simulink model "soce"  (R2024a)
settings: Solver=VariableStepAuto  StartTime=0.0  StopTime=10  FixedStep=500e-6  RelTol=1e-3
values from neighbouring files (symbols this model uses):
  C1_pack = C1 * parallel_cells / series_cells    (= 0.0780484375)    [soc.m]
  C2_pack = C2 * parallel_cells / series_cells    (= 0.0972984375)    [soc.m]
  internal_resistance_pack = int_cell_resistance * series_cells / parallel_cells + electronic_resistance    (= 0.104737272727)    [soc.m]
  Q_2RC = 1    [soc.m]
  R = [sigma_V^2, 0 ... (first row only)    [soc.m]
  R1_pack = R1 * series_cells / parallel_cells    (= 0.0116363636364)    [soc.m]
  R2_pack = R2 * series_cells / parallel_cells    (= 0.0116363636364)    [soc.m]
undefined symbols (not defined in the file or in its folder): rated_cell_capacity, T_vec
libraries: simulink x10, spsVariableCapacitorLib x3, spsVariableResistorLib x3, spsCurrentMeasurementLib x2, spsVoltageMeasurementLib x2, spsControlledVoltageSourceLib x1, spsControlledCurrentSourceLib x1, sps_lib x1
settings Model: Creator=DELL  LastModifiedBy=DELL

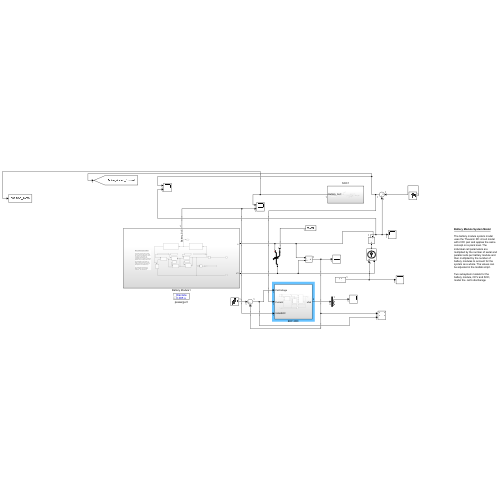
[thumbnail: Simulink's stored preview of the top-level diagram]
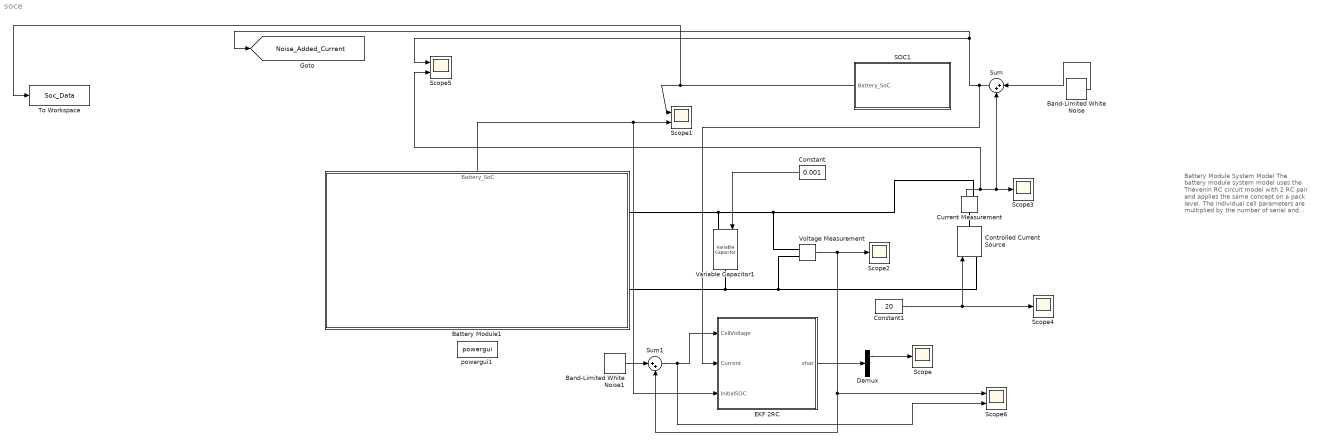
== system soce ==
  note: Battery Module System Model
      |
      | The battery module system model uses the Thevenin RC circuit model with 2 RC pair and applies the same concept on a pack level. The individual cell parameters are multiplied by the number of serial and parallel cells per battery module and then multiplied by the number of battery module s to account for the system as a whole. The values can be adjusted in the matlab script.
      |
      | Two subsystem models for the battery module , OCV and SOC, model the cell's discharage characteristic and state of charge for the ESUs.
  Band-Limited White Noise : simulink/Sources/Band-Limited White Noise  Cov=0  Ts=1  seed=12345
  Band-Limited White Noise1 : simulink/Sources/Band-Limited White Noise  Cov=0  Ts=0.01  seed=12345
  Battery Module1 : Subsystem
      settings: PortSchema="{\"entries\":[{\"content\":{\"sides\":[{\"content\":{},\"type\":\"ConnectorPlacement.EquallySpacedRectSide\",\"uuid\":\"1cf2e637-c056-448b-9d8f-ed664b461c4e\"},{\"content\":{\"connectorIds\":[\"RConn1\",\"RConn2\"],\"side\":\"RIGHT\"},\"type\":\"ConnectorPlacement.EquallySpacedRectSide\",\"uuid\":\"9015fd1e-0347-435a-aa67-edb519119c95\"},{\"content\":{\"connectorIds\":[\"Out1\"],\"side\":\"TOP\"},\"type\":\"ConnectorPlacement.EquallySpacedRectSide\",\"uuid\":\"8eddc867-8dee-40eb-ad4a-8474d27a660f\"}]},\"type\":\"ConnectorPlacement.EquallySpacedConnector\",\"uuid\":\"c8be1dcd-ca4d-45ed-81e7-8f26517ac315\"}],\"packageUris\":[\"http://schema.mathworks.com/mf0/Connector/R2020b\"],\"version\":\"1.0\"}"
  Constant : Constant  Value=0.001
  Constant1 : Constant  Value=20
  Controlled Current Source : spsControlledCurrentSourceLib/Controlled Current Source  Initialize=on  Source_Type=AC  Amplitude=0  Phase=0  Frequency=0  Measurements=None
  Current Measurement : spsCurrentMeasurementLib/Current Measurement  PhasorSimulation=off  OutputType=Complex  PSBequivalent=0
  Demux : Demux  Outputs=3
  EKF 2RC : Subsystem  VariantControl=EKF 2RC
      settings: LibrarySourceBlock=|
      | BatteryEstimators/SOC Estimator
      | (Kalman Filter)/Kalman Filter/EKF 2RC
  SOC1 : Subsystem
  Scope{,2..4} (4 alike) : Scope
  Scope1 : Scope  NumInputPorts=2
  Scope5 : Scope  NumInputPorts=2
  Scope6 : Scope  NumInputPorts=2
  Sum : Sum  Inputs=|++
  Sum1 : Sum  Inputs=|++
  To Workspace : ToWorkspace  VariableName=Soc_Data  SaveFormat=Timeseries  SampleTime=-1
  Variable Capacitor1 : spsVariableCapacitorLib/Variable Capacitor  methode=Backward Euler  Cabsmin=1e-9  Initialize=on  vC0=0.001  C0=1e-6  iC0=0
      settings: LibrarySourceBlock=sps_lib/Passives/Variable Capacitor
  Voltage Measurement : spsVoltageMeasurementLib/Voltage Measurement  PhasorSimulation=off  OutputType=Complex  PSBequivalent=0
  powergui1 : sps_lib/powergui  SimulationMode=Discrete  SampleTime=0.005  frequency=60  Iterations=50  frequencyindice=0  Pbase=100e6  ErrMax=1e-4  UnitsV=kV  UnitsW=MW  buscounter=0  FunctionMessages=off  echomessages=off  EnableUseOfTLC=off  CurrentSourceSwitches=off  DisableSnubberDevices=off  DisableRonSwitches=off  DisableVfSwitches=off  DisplayEquations=off  AutomaticDiscreteSolvers=off  SolverType=Tustin  Interpol=off  ExternalGateDelay=off  methode=off  Ts=0  x0status=blocks  SPID=off  SwTol=0  HookPort=off  NonlinearTolerance=1e-4  nMaxIteration=100  ContinueOnMaxIteration=off  RestoreLinks=warning  ResistiveCurrentMeasurement=off  Frange=[0:2:500]  Ylog=off  Xlog=on  ShowGrid=off  save=off  variable=ZData  structure=0  ZoomFFT=on  StartTime=0.0  cycles=1  DisplayStyle=1  fundamental=60  FreqAxis=off  MaxFrequency=1000  frequencyindicesteady=1  RmsSteady=1  display=off
  tag scope: Noise_Added_Current=global
  wires:
  Band-Limited White Noise/1 -> Sum/1
  SOC1/1(Battery_SoC) -> To Workspace/1, Scope1/1
  Constant/1 -> Variable Capacitor1/1
  Current Measurement/1 -> Scope3/1, Sum/2, Scope5/2
  Constant1/1 -> Scope4/1, Controlled Current Source/1
  Band-Limited White Noise1/1 -> Sum1/1
  Sum/1 -> EKF 2RC/2(Current), Scope5/1, [Noise_Added_Current]
  Voltage Measurement/1 -> Scope2/1, Sum1/2, Scope6/1
  Battery Module1/1(Battery_SoC) -> EKF 2RC/3(InitialSOC), Scope1/2
  Sum1/1 -> Scope6/2, EKF 2RC/1(CellVoltage)
  EKF 2RC/1(xhat) -> Demux/1
  Demux/1 -> Scope/1
  connections:
  Variable Capacitor1/LConn1 -- Battery Module1/RConn1 -- Voltage Measurement/LConn2 -- Current Measurement/RConn1
  Controlled Current Source/LConn1 -- Voltage Measurement/LConn1 -- Battery Module1/RConn2 -- Variable Capacitor1/RConn1
  Current Measurement/LConn1 -- Controlled Current Source/RConn1

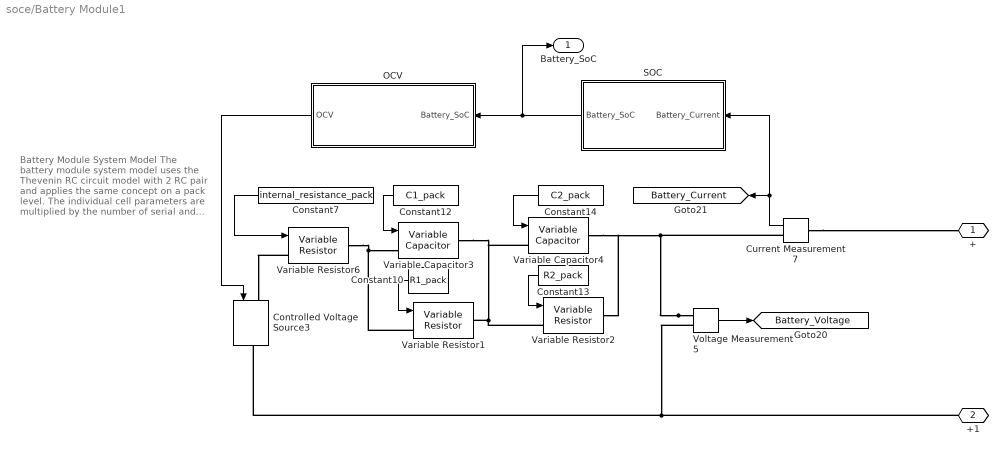
== system soce/Battery Module1 ==
  note: Battery Module System Model
      |
      | The battery module system model uses the Thevenin RC circuit model with 2 RC pair and applies the same concept on a pack level. The individual cell parameters are multiplied by the number of serial and parallel cells per battery module and then multiplied by the number of battery modules to account for the system as a whole. The values can be adjusted in the matlab script.
      |
      | Two subsystem models for the battery module, OCV and SOC, model the cell's discharage characteristic and state of charge for the ESUs.
  Constant10 : Constant  Value=R1_pack
  Constant12 : Constant  Value=C1_pack
  Constant13 : Constant  Value=R2_pack
  Constant14 : Constant  Value=C2_pack
  Constant7 : Constant  Value=internal_resistance_pack
  Controlled Voltage Source3 : spsControlledVoltageSourceLib/Controlled Voltage Source  Initialize=on  Source_Type=DC  Amplitude=537.6  Phase=0  Frequency=1  Measurements=None
  Current Measurement7 : spsCurrentMeasurementLib/Current Measurement  PhasorSimulation=off  OutputType=Complex  PSBequivalent=0
  OCV : Subsystem
  SOC : Subsystem
  Variable Capacitor3 : spsVariableCapacitorLib/Variable Capacitor  methode=Backward Euler  Cabsmin=1e-9  Initialize=off  vC0=4  C0=6  iC0=0
  Variable Capacitor4 : spsVariableCapacitorLib/Variable Capacitor  methode=Backward Euler  Cabsmin=1e-9  Initialize=off  vC0=0  C0=1100e-3  iC0=0
  Variable Resistor1 : spsVariableResistorLib/Variable Resistor  Rabsmin=1e-3
  Variable Resistor2 : spsVariableResistorLib/Variable Resistor  Rabsmin=1e-3
  Variable Resistor6 : spsVariableResistorLib/Variable Resistor  Rabsmin=1e-3
      settings: LibrarySourceBlock=sps_lib/Passives/Variable Resistor
  Voltage Measurement5 : spsVoltageMeasurementLib/Voltage Measurement  PhasorSimulation=off  OutputType=Complex  PSBequivalent=0
  + : PMIOPort  Side=Right
  +1 : PMIOPort  Port=2  Side=Right
  Battery_SoC : Outport
  tag scope: Battery_Current=global, Battery_Voltage=global
  wires:
  OCV/1(OCV) -> Controlled Voltage Source3/1
  Voltage Measurement5/1 -> [Battery_Voltage]
  Current Measurement7/1 -> SOC/1(Battery_Current), [Battery_Current]
  SOC/1(Battery_SoC) -> Battery_SoC/1, OCV/1(Battery_SoC)
  Constant14/1 -> Variable Capacitor4/1
  Constant7/1 -> Variable Resistor6/1
  Constant12/1 -> Variable Capacitor3/1
  Constant10/1 -> Variable Resistor1/1
  Constant13/1 -> Variable Resistor2/1
  connections:
  Variable Resistor2/LConn1 -- Variable Capacitor4/LConn1 -- Variable Capacitor3/RConn1 -- Variable Resistor1/RConn1
  Variable Resistor1/LConn1 -- Variable Resistor6/RConn1 -- Variable Capacitor3/LConn1
  Voltage Measurement5/LConn1 -- +1/RConn1 -- Controlled Voltage Source3/RConn1
  Variable Resistor6/LConn1 -- Controlled Voltage Source3/LConn1
  Voltage Measurement5/LConn2 -- Variable Resistor2/RConn1 -- Variable Capacitor4/RConn1 -- Current Measurement7/RConn1
  Current Measurement7/LConn1 -- +/RConn1

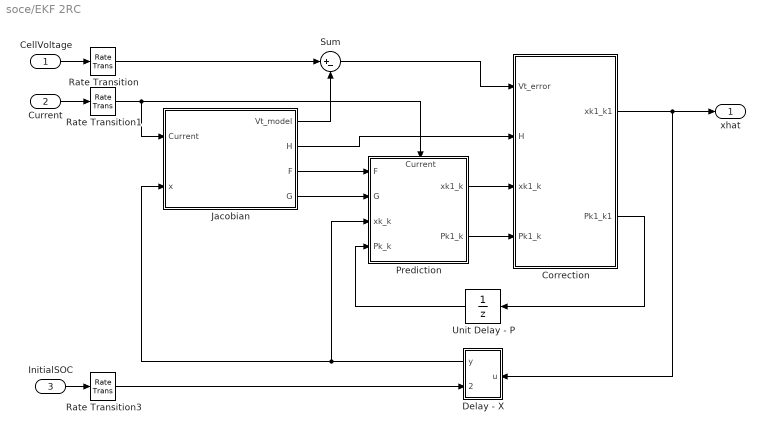
== system soce/EKF 2RC ==
  CellVoltage : Inport
  Current : Inport  Port=2
  InitialSOC : Inport  Port=3
  Correction : Subsystem
  Delay - X : Subsystem
      settings: PortSchema="{\"entries\":[{\"content\":{\"sides\":[{\"content\":{\"connectorIds\":[\"In1\"]},\"type\":\"ConnectorPlacement.EquallySpacedRectSide\",\"uuid\":\"3362b6e3-9ef0-414f-8c36-2f543f704d9c\"},{\"content\":{\"connectorIds\":[\"Out1\",\"In2\"],\"side\":\"RIGHT\"},\"type\":\"ConnectorPlacement.EquallySpacedRectSide\",\"uuid\":\"11e7d0c5-4a27-4b8c-b505-ab30596c2b25\"},{\"content\":{\"connectorIds\":[],\"side\":\"TOP\"},\"type\":\"ConnectorPlacement.EquallySpacedRectSide\",\"uuid\":\"2d2b4d79-d4b9-4064-9377-c3a75a280e90\"}]},\"type\":\"ConnectorPlacement.EquallySpacedConnector\",\"uuid\":\"61e54eb8-002c-4ced-aad8-a34ad65d09af\"}],\"packageUris\":[\"http://schema.mathworks.com/mf0/Connector/R2020b\"],\"version\":\"1.0\"}"
  Jacobian : Subsystem
  Prediction : Subsystem
      settings: PortSchema="{\"entries\":[{\"content\":{\"sides\":[{\"content\":{\"connectorIds\":[\"In1\",\"In2\",\"In3\",\"In4\"]},\"type\":\"ConnectorPlacement.EquallySpacedRectSide\",\"uuid\":\"769ad24d-2d7f-40f9-a049-32dd41bae35d\"},{\"content\":{\"connectorIds\":[\"Out1\",\"Out2\"],\"side\":\"RIGHT\"},\"type\":\"ConnectorPlacement.EquallySpacedRectSide\",\"uuid\":\"b91eca28-d625-4904-9292-6163fd48fb7b\"},{\"content\":{\"connectorIds\":[\"In5\"],\"side\":\"TOP\"},\"type\":\"ConnectorPlacement.EquallySpacedRectSide\",\"uuid\":\"03f245fa-72f0-4cdc-a162-c307173ac60c\"}]},\"type\":\"ConnectorPlacement.EquallySpacedConnector\",\"uuid\":\"70aef080-af31-4b50-8c38-7ffc1907abe4\"}],\"packageUris\":[\"http://schema.mathworks.com/mf0/Connector/R2020b\"],\"version\":\"1.0\"}"
  Rate Transition : RateTransition
  Rate Transition1 : RateTransition
  Rate Transition3 : RateTransition
  Sum : Sum  Inputs=|+-
  Unit Delay - P : UnitDelay  SampleTime=-1  HasFrameUpgradeWarning=on
  xhat : Outport
  wires:
  Current/1 -> Rate Transition1/1
  Prediction/1(xk1_k) -> Correction/3(xk1_k)
  Jacobian/1(Vt_model) -> Sum/2
  Rate Transition3/1 -> Delay - X/2(SOC0)
  CellVoltage/1 -> Rate Transition/1
  Rate Transition1/1 -> Prediction/5(Current), Jacobian/1(Current)
  Sum/1 -> Correction/1(Vt_error)
  Jacobian/4(G) -> Prediction/2(G)
  Correction/2(Pk1_k1) -> Unit Delay - P/1
  Delay - X/1(y) -> Prediction/3(xk_k), Jacobian/2(x)
  Prediction/2(Pk1_k) -> Correction/4(Pk1_k)
  Jacobian/2(H) -> Correction/2(H)
  Rate Transition/1 -> Sum/1
  Correction/1(xk1_k1) -> xhat/1, Delay - X/1(u)
  Unit Delay - P/1 -> Prediction/4(Pk_k)
  Jacobian/3(F) -> Prediction/1(F)
  InitialSOC/1 -> Rate Transition3/1

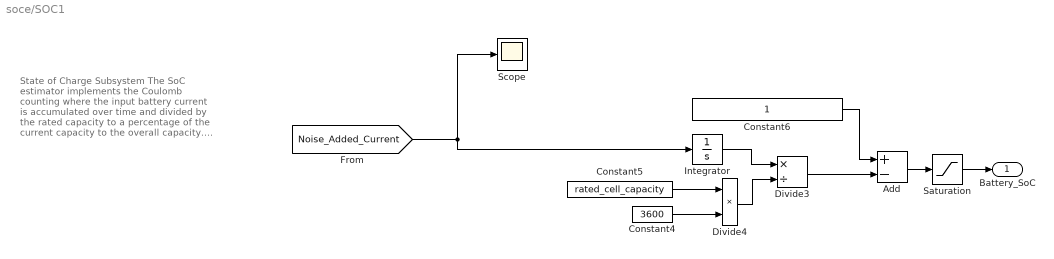
== system soce/SOC1 ==
  note: State of Charge Subsystem
      |
      | The SoC estimator implements the Coulomb counting where the input battery current is accumulated over time and divided by the rated capacity to a percentage of the current capacity to the overall capacity. The output of this subsystem outputs the state of charge as a percentage.
  Add : Sum  Inputs=+-
  Constant4 : Constant  Value=3600
  Constant5 : Constant  Value=rated_cell_capacity
  Constant6 : Constant
  Divide3 : Product  Inputs=*/
  Divide4 : Product  Inputs=**
  Integrator : Integrator
  Saturation : Saturate  UpperLimit=1  LowerLimit=0
  Scope : Scope
  Battery_SoC : Outport
  wires:
  Constant6/1 -> Add/1
  Divide3/1 -> Add/2
  Divide4/1 -> Divide3/2
  Constant5/1 -> Divide4/1
  Integrator/1 -> Divide3/1
  Constant4/1 -> Divide4/2
  [Noise_Added_Current] -> Integrator/1, Scope/1
  Saturation/1 -> Battery_SoC/1
  Add/1 -> Saturation/1

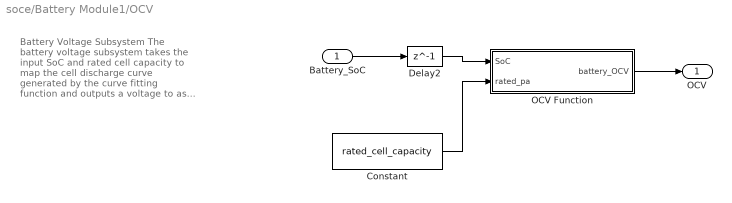
== system soce/Battery Module1/OCV ==
  note: Battery Voltage Subsystem
      |
      | The battery voltage subsystem takes the input SoC and rated cell capacity to map the cell discharge curve generated by the curve fitting function and outputs a voltage to as an input to the voltage source.
  Battery_SoC : Inport
  Constant : Constant  Value=rated_cell_capacity
  Delay2 : Delay  DelayLength=1  InitialCondition=1
  OCV Function : MATLAB Function  TreatAsAtomicUnit=on
  OCV : Outport
  wires:
  Delay2/1 -> OCV Function/1(SoC)
  OCV Function/1(battery_OCV) -> OCV/1
  Battery_SoC/1 -> Delay2/1
  Constant/1 -> OCV Function/2(rated_pa)

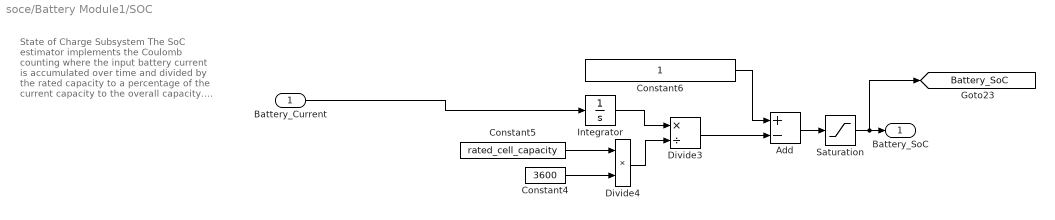
== system soce/Battery Module1/SOC ==
  note: State of Charge Subsystem
      |
      | The SoC estimator implements the Coulomb counting where the input battery current is accumulated over time and divided by the rated capacity to a percentage of the current capacity to the overall capacity. The output of this subsystem outputs the state of charge as a percentage.
  Battery_Current : Inport
  Add : Sum  Inputs=+-
  Constant4 : Constant  Value=3600
  Constant5 : Constant  Value=rated_cell_capacity
  Constant6 : Constant
  Divide3 : Product  Inputs=*/
  Divide4 : Product  Inputs=**
  Integrator : Integrator
  Saturation : Saturate  UpperLimit=1  LowerLimit=0
  Battery_SoC : Outport
  tag scope: Battery_SoC=global
  wires:
  Constant6/1 -> Add/1
  Divide3/1 -> Add/2
  Divide4/1 -> Divide3/2
  Constant5/1 -> Divide4/1
  Integrator/1 -> Divide3/1
  Constant4/1 -> Divide4/2
  Battery_Current/1 -> Integrator/1
  Saturation/1 -> [Battery_SoC], Battery_SoC/1
  Add/1 -> Saturation/1

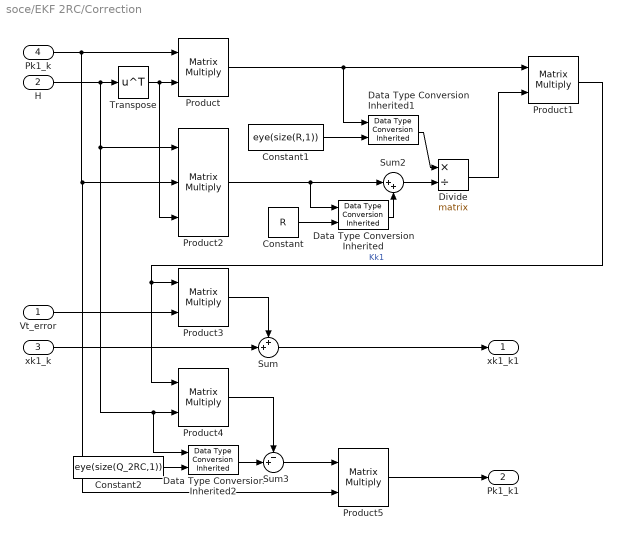
== system soce/EKF 2RC/Correction ==
  Vt_error : Inport
  H : Inport  Port=2
  xk1_k : Inport  Port=3
  Pk1_k : Inport  Port=4
  Constant : Constant  Value=R
  Constant1 : Constant  Value=eye(size(R,1))
  Constant2 : Constant  Value=eye(size(Q_2RC,1))
  Data Type Conversion Inherited : simulink/Signal Attributes/Data Type Conversion Inherited  ConvertRealWorld=Real World Value  DoSatur=off
  Data Type Conversion Inherited1 : simulink/Signal Attributes/Data Type Conversion Inherited  ConvertRealWorld=Real World Value  DoSatur=off
  Data Type Conversion Inherited2 : simulink/Signal Attributes/Data Type Conversion Inherited  ConvertRealWorld=Real World Value  DoSatur=off
  Divide : Product  Inputs=*/  Multiplication=Matrix(*)
  Product{,1,3..5} (5 alike) : Product  Multiplication=Matrix(*)
  Product2 : Product  Inputs=3  Multiplication=Matrix(*)
  Sum : Sum  Inputs=++|
  Sum2 : Sum  Inputs=|++
  Sum3 : Sum  Inputs=-+|
  Transpose : Math  Operator=transpose
  xk1_k1 : Outport
  Pk1_k1 : Outport  Port=2
  wires:
  Product5/1 -> Pk1_k1/1
  Sum3/1 -> Product5/1
  Product4/1 -> Sum3/1
  Sum/1 -> xk1_k1/1
  Product3/1 -> Sum/1
  Vt_error/1 -> Product3/2
  xk1_k/1 -> Sum/2
  Divide/1 -> Product1/2
  Sum2/1 -> Divide/2
  Product1/1 -> Product3/1, Product4/1  "Kk1"
  Product2/1 -> Data Type Conversion Inherited/1, Sum2/1
  Product/1 -> Data Type Conversion Inherited1/1, Product1/1
  Pk1_k/1 -> Product/1, Product2/2, Product5/2
  Transpose/1 -> Product/2, Product2/3
  H/1 -> Transpose/1, Product2/1, Data Type Conversion Inherited2/1, Product4/2
  Data Type Conversion Inherited/1 -> Sum2/2
  Constant/1 -> Data Type Conversion Inherited/2
  Data Type Conversion Inherited1/1 -> Divide/1
  Constant1/1 -> Data Type Conversion Inherited1/2
  Data Type Conversion Inherited2/1 -> Sum3/2
  Constant2/1 -> Data Type Conversion Inherited2/2

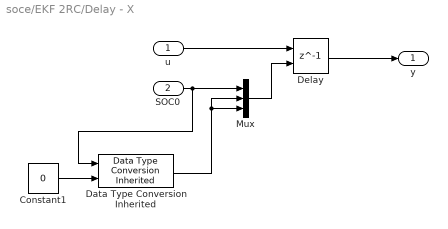
== system soce/EKF 2RC/Delay - X ==
  u : Inport
  SOC0 : Inport  Port=2
  Constant1 : Constant  Value=0
  Data Type Conversion Inherited : simulink/Signal Attributes/Data Type Conversion Inherited  ConvertRealWorld=Real World Value  DoSatur=off
  Delay : Delay  DelayLength=1  InitialConditionSource=Input port
      settings: InputPortMap=u0,p4
  Mux : Mux  Inputs=3
  y : Outport
  wires:
  u/1 -> Delay/1
  Delay/1 -> y/1
  Mux/1 -> Delay/2
  SOC0/1 -> Data Type Conversion Inherited/1, Mux/1
  Data Type Conversion Inherited/1 -> Mux/2, Mux/3
  Constant1/1 -> Data Type Conversion Inherited/2

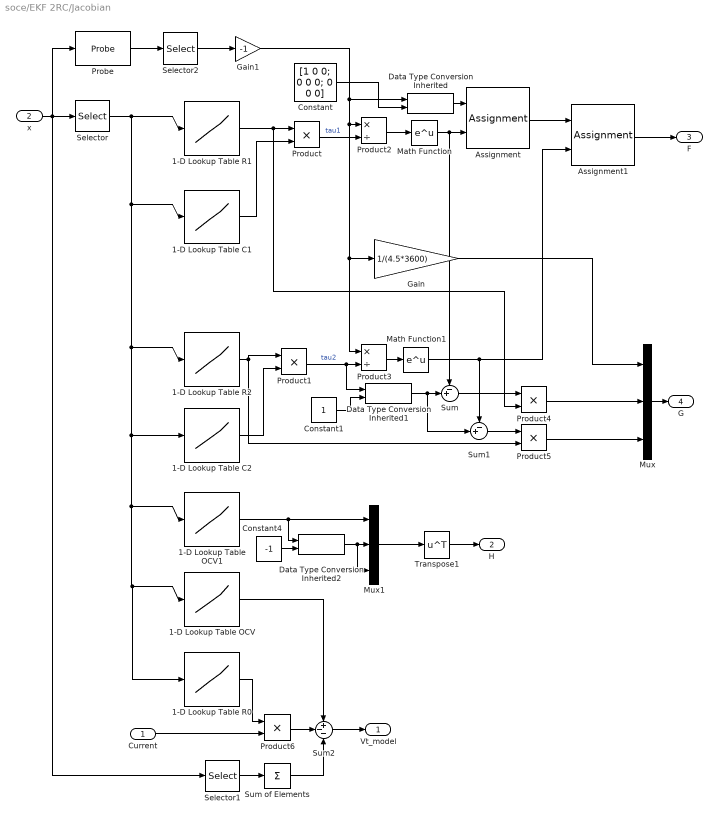
== system soce/EKF 2RC/Jacobian ==
  Current : Inport
  x : Inport  Port=2
  1-D Lookup Table C1 : Lookup_n-D  NumberOfTableDimensions=1  BreakpointsForDimension1=[0,10,20,30,40,50,60,70,80,90,100]  BreakpointsForDimension2=T_vec  Table=[1000,1100,1200,1300,1400,1500,1600,1700,1800,1900,2000]  InternalRulePriority=Speed  RndMeth=Simplest
  1-D Lookup Table C2 : Lookup_n-D  NumberOfTableDimensions=1  BreakpointsForDimension1=[10,20,30,40,50,60,70,80,90,100]  BreakpointsForDimension2=T_vec  Table=[500,550,600,650,700,750,800,850,900,950]  InternalRulePriority=Speed  RndMeth=Simplest
  1-D Lookup Table OCV : Lookup_n-D  NumberOfTableDimensions=1  BreakpointsForDimension1=[10,20,30,40,50,60,70,80,90,100]  BreakpointsForDimension2=T_vec  Table=[3.2,3.3,3.4,3.5,3.6,3.7,3.8,3.9,4.0,4.1]  InternalRulePriority=Speed  RndMeth=Simplest
  1-D Lookup Table OCV1 : Lookup_n-D  NumberOfTableDimensions=1  BreakpointsForDimension1=[10,20,30,40,50,60,70,80,90,100]  BreakpointsForDimension2=T_vec  Table=[0.05,0.04,0.04,0.03,0.02,0.02,0.02,0.01,0.01,0.00]  InternalRulePriority=Speed  RndMeth=Simplest
  1-D Lookup Table R0 : Lookup_n-D  NumberOfTableDimensions=1  BreakpointsForDimension1=[0,10,20,30,40,50,60,70,80,90,100]  BreakpointsForDimension2=T_vec  Table=[0.05,0.045,0.04,0.035,0.03,0.025,0.02,0.015,0.01,0.005,0.001]  InternalRulePriority=Speed  RndMeth=Simplest
  1-D Lookup Table R1 : Lookup_n-D  NumberOfTableDimensions=1  BreakpointsForDimension1=[0,10,20,30,40,50,60,70,80,90,100]  BreakpointsForDimension2=T_vec  Table=[0.02,0.018,0.016,0.014,0.012,0.01,0.008,0.006,0.004,0.002,0.001]  InternalRulePriority=Speed  RndMeth=Simplest
  1-D Lookup Table R2 : Lookup_n-D  NumberOfTableDimensions=1  BreakpointsForDimension1=[0,10,20,30,40,50,60,70,80,90,100]  BreakpointsForDimension2=T_vec  Table=[0.05,0.045,0.04,0.035,0.03,0.025,0.02,0.015,0.01,0.005,0.001]  InternalRulePriority=Speed  RndMeth=Simplest
  Assignment : Assignment  NumberOfDimensions=2  DiagnosticForDimensions=Warning  IndexOptions=Index vector (dialog),Index vector (dialog)  Indices=2,2  OutputSizes=1,1
  Assignment1 : Assignment  NumberOfDimensions=2  DiagnosticForDimensions=Warning  IndexOptions=Index vector (dialog),Index vector (dialog)  Indices=3,3  OutputSizes=1,1
  Constant : Constant  Value=|
      | [1 0  0;
      | 0 0 0;
      | 0 0 0]
  Constant1 : Constant
  Constant4 : Constant  Value=-1
  Data Type Conversion Inherited : simulink/Signal Attributes/Data Type Conversion Inherited  ConvertRealWorld=Real World Value  DoSatur=off
  Data Type Conversion Inherited1 : simulink/Signal Attributes/Data Type Conversion Inherited  ConvertRealWorld=Real World Value  DoSatur=off
  Data Type Conversion Inherited2 : simulink/Signal Attributes/Data Type Conversion Inherited  ConvertRealWorld=Real World Value  DoSatur=off
  Gain : Gain  Gain=1/(4.5*3600)
  Gain1 : Gain  Gain=-1
  Math Function : Math
  Math Function1 : Math
  Mux : Mux  Inputs=3
  Mux1 : Mux  Inputs=3
  Probe : Probe  ProbeWidth=off  ProbeComplexSignal=off  ProbeSampleTimeDataType=Same as input
  Product{,1,4..6} (5 alike) : Product
  Product2 : Product  Inputs=*/
  Product3 : Product  Inputs=*/
  Selector : Selector  InputPortWidth=3  IndexOptions=Index vector (dialog)  Indices=1  OutputSizes=1
  Selector1 : Selector  InputPortWidth=3  IndexOptions=Index vector (dialog)  Indices=[2 3]  OutputSizes=1
  Selector2 : Selector  InputPortWidth=2  IndexOptions=Index vector (dialog)  Indices=1  OutputSizes=1
  Sum : Sum  Inputs=-+|
  Sum of Elements : Sum  Inputs=+
  Sum1 : Sum  Inputs=-+|
  Sum2 : Sum  Inputs=+--
  Transpose1 : Math  Operator=transpose
  Vt_model : Outport
  H : Outport  Port=2
  F : Outport  Port=3
  G : Outport  Port=4
  wires:
  Selector2/1 -> Gain1/1
  Probe/1 -> Selector2/1
  Gain/1 -> Mux/1
  Selector/1 -> 1-D Lookup Table R1/1, 1-D Lookup Table C1/1, 1-D Lookup Table R2/1, 1-D Lookup Table C2/1, 1-D Lookup Table OCV1/1, 1-D Lookup Table OCV/1, 1-D Lookup Table R0/1
  1-D Lookup Table OCV1/1 -> Data Type Conversion Inherited2/1, Mux1/1
  1-D Lookup Table OCV/1 -> Sum2/1
  Sum2/1 -> Vt_model/1
  Transpose1/1 -> H/1
  Mux1/1 -> Transpose1/1
  Current/1 -> Product6/2
  Sum of Elements/1 -> Sum2/3
  Selector1/1 -> Sum of Elements/1
  Product6/1 -> Sum2/2
  1-D Lookup Table R0/1 -> Product6/1
  Mux/1 -> G/1
  Product5/1 -> Mux/3
  Product4/1 -> Mux/2
  Gain1/1 -> Data Type Conversion Inherited/1, Product2/1, Gain/1, Product3/1
  Sum1/1 -> Product5/1
  Sum/1 -> Product4/1
  Assignment1/1 -> F/1
  Product3/1 -> Math Function1/1
  Product2/1 -> Math Function/1
  Product1/1 -> Data Type Conversion Inherited1/1, Product3/2  "tau2"
  Product/1 -> Product2/2  "tau1"
  1-D Lookup Table C2/1 -> Product1/2
  1-D Lookup Table R2/1 -> Product5/2, Product1/1
  1-D Lookup Table C1/1 -> Product/2
  1-D Lookup Table R1/1 -> Product/1, Product4/2
  Math Function/1 -> Sum/1, Assignment/2
  Math Function1/1 -> Assignment1/2, Sum1/1
  Assignment/1 -> Assignment1/1
  x/1 -> Selector/1, Selector1/1, Probe/1
  Data Type Conversion Inherited/1 -> Assignment/1
  Constant/1 -> Data Type Conversion Inherited/2
  Data Type Conversion Inherited1/1 -> Sum1/2, Sum/2
  Constant1/1 -> Data Type Conversion Inherited1/2
  Constant4/1 -> Data Type Conversion Inherited2/2
  Data Type Conversion Inherited2/1 -> Mux1/3, Mux1/2

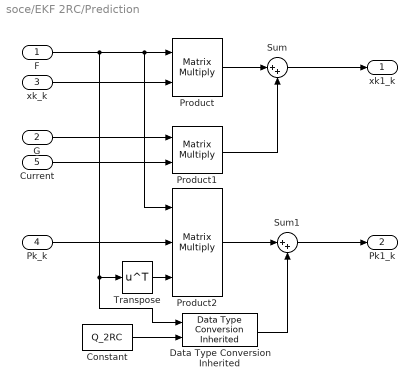
== system soce/EKF 2RC/Prediction ==
  F : Inport
  G : Inport  Port=2
  xk_k : Inport  Port=3
  Pk_k : Inport  Port=4
  Current : Inport  Port=5
  Constant : Constant  Value=Q_2RC
  Data Type Conversion Inherited : simulink/Signal Attributes/Data Type Conversion Inherited  ConvertRealWorld=Real World Value  DoSatur=off
  Product : Product  Multiplication=Matrix(*)
  Product1 : Product  Multiplication=Matrix(*)
  Product2 : Product  Inputs=3  Multiplication=Matrix(*)
  Sum : Sum  Inputs=|++
  Sum1 : Sum  Inputs=|++
  Transpose : Math  Operator=transpose
  xk1_k : Outport
  Pk1_k : Outport  Port=2
  wires:
  Sum1/1 -> Pk1_k/1
  Product2/1 -> Sum1/1
  Transpose/1 -> Product2/3
  Pk_k/1 -> Product2/2
  Sum/1 -> xk1_k/1
  Product1/1 -> Sum/2
  Product/1 -> Sum/1
  Current/1 -> Product1/2
  G/1 -> Product1/1
  xk_k/1 -> Product/2
  F/1 -> Product/1, Product2/1, Data Type Conversion Inherited/1, Transpose/1
  Data Type Conversion Inherited/1 -> Sum1/2
  Constant/1 -> Data Type Conversion Inherited/2

== matlab function soce/Battery Module1/OCV/OCV Function ==
  data: SoC input; battery_OCV output; rated_pa input
function battery_OCV = OCV(SoC,rated_pa)
%0.7813   -5.9896   12.2396  -10.1354    4.4342    2.8500
SoC=rated_pa-SoC*rated_pa;

%LG Cell coefficients
% a_ocv= -0.0399;
% b_ocv= 0.2547;
% c_ocv= -0.5498;
% d_ocv= 0.4558;
% e_ocv= -0.3859;
% f_ocv= 4.1677;

%Murata cell VTC6 coefficient
% a_ocv= -0.0745;
% b_ocv= 0.4871;
% c_ocv= -1.1206;
% d_ocv= 1.0556;
% e_ocv= -0.6461;
% f_ocv= 4.1708;

% %Molicell P28A
% a_ocv= -0.1386;
% b_ocv= 0.8289;
% c_ocv= -1.7437;
% d_ocv= 1.5487;
% e_ocv= -0.8711;
% f_ocv= 4.1867;

%Molicell P45B
a_ocv= -0.0090;
b_ocv= 0.0876;
c_ocv= -0.3010;
d_ocv= 0.4144;
e_ocv= -0.3841;
f_ocv= 4.1717;

cell_voltage = a_ocv*SoC.^5 + b_ocv*SoC.^4 + c_ocv*SoC.^3 + d_ocv*SoC.^2 + e_ocv*SoC + f_ocv;

%cell_voltage =  -1.031*exp(-35*SoC)+3.685+0.2156*SoC-0.1178*SoC.^2+.3201*SoC.^3;

%cell_voltage = a_ocv*exp(b_ocv*SoC)+c_ocv*exp(d_ocv*SoC)+e_ocv*SoC^2;
battery_OCV = cell_voltage;

% a_ocv= 3.289;
% b_ocv= 1.137;
% c_ocv= 0.8287;
% d_ocv= -10.31;
% e_ocv= -10.04;
